simulink model "Leg_vmc_simu"  (R2021a)
settings: Solver=VariableStepAuto  StartTime=0.0  StopTime=10.0  RelTol=1e-3
undefined symbols (not defined in the file): c1, c2, coef, D, g, I_x, k1, k2, M
settings Model: Creator=solitude  LastModifiedBy=MSI_NB
settings SolverCC: AlgebraicLoopSolver=TrustRegion
settings DebuggingCC: SFMachineParentedDataDiag=warning

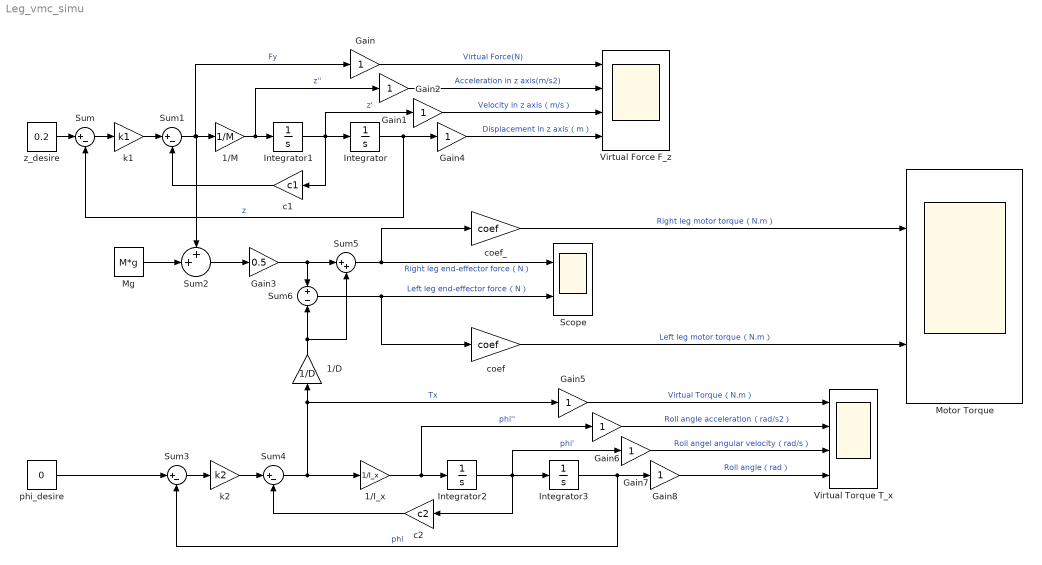
== system Leg_vmc_simu ==
  1/D : Gain  Gain=1/D
  "1/I_x " : Gain  Gain=1/I_x
  1/M : Gain  Gain=1/M
  Gain{,1..2,4..8} (8 alike) : Gain
  Gain3 : Gain  Gain=0.5
  Integrator : Integrator
  Integrator1 : Integrator
  Integrator2 : Integrator
  Integrator3 : Integrator  InitialCondition=0.2
  Mg : Constant  Value=M*g
  Motor Torque : Scope  NumInputPorts=2
  Scope : Scope  NumInputPorts=2
  Sum{,1,3..4} (4 alike) : Sum  Inputs=|+-
  Sum2 : Sum  Inputs=++|
  Sum5 : Sum  Inputs=|++
  Sum6 : Sum  Inputs=+|-
  Virtual Force F_z : Scope  NumInputPorts=4
  Virtual Torque T_x : Scope  NumInputPorts=4
  c1 : Gain  Gain=c1
  c2 : Gain  Gain=c2
  coef : Gain  Gain=coef
  coef_ : Gain  Gain=coef
  k1 : Gain  Gain=k1
  k2 : Gain  Gain=k2
  phi_desire : Constant  Value=0
  z_desire : Constant  Value=0.2
  wires:
  z_desire/1 -> Sum/1
  1/M/1 -> Integrator1/1, Gain1/1  "z''"
  Integrator1/1 -> c1/1, Gain2/1, Integrator/1  "z'"
  Integrator/1 -> Gain4/1, Sum/2  "z"
  Sum/1 -> k1/1
  k1/1 -> Sum1/1
  c1/1 -> Sum1/2
  Sum1/1 -> 1/M/1, Sum2/1, Gain/1  "Fy"
  Mg/1 -> Sum2/2
  Sum2/1 -> Gain3/1
  phi_desire/1 -> Sum3/1
  Sum3/1 -> k2/1
  k2/1 -> Sum4/1
  Sum4/1 -> "1/I_x "/1, Gain5/1, 1/D/1  "Tx"
  "1/I_x "/1 -> Integrator2/1, Gain6/1  "phi''"
  Integrator2/1 -> c2/1, Gain7/1, Integrator3/1  "phi'"
  Integrator3/1 -> Gain8/1, Sum3/2  "phi"
  c2/1 -> Sum4/2
  Gain3/1 -> Sum6/1, Sum5/1
  Sum5/1 -> Scope/1, coef_/1  "Right leg end-effector force（N）"
  Sum6/1 -> coef/1, Scope/2  "Left leg end-effector force（N）"
  1/D/1 -> Sum5/2, Sum6/2
  coef_/1 -> Motor Torque/1  "Right leg motor torque（N.m）"
  coef/1 -> Motor Torque/2  "Left leg motor torque（N.m）"
  Gain/1 -> Virtual Force F_z/1  "Virtual Force(N)"
  Gain1/1 -> Virtual Force F_z/2  "Acceleration in z axis(m/s2)"
  Gain2/1 -> Virtual Force F_z/3  "Velocity in z axis（m/s）"
  Gain4/1 -> Virtual Force F_z/4  "Displacement in z axis（m）"
  Gain5/1 -> Virtual Torque T_x/1  "Virtual Torque（N.m）"
  Gain6/1 -> Virtual Torque T_x/2  "Roll angle acceleration（rad/s2）"
  Gain7/1 -> Virtual Torque T_x/3  "Roll angel angular velocity（rad/s）"
  Gain8/1 -> Virtual Torque T_x/4  "Roll angle（rad）"
